simulink model "doublePendulum"  (R2022a)
settings: Solver=ode45  StartTime=0.0  StopTime=50  MaxStep=0.001  RelTol=1e-4
undefined symbols (not defined in the file): a_x, a_y, omega_x, omega_y
settings Model: Creator=semen  LastModifiedBy=semen

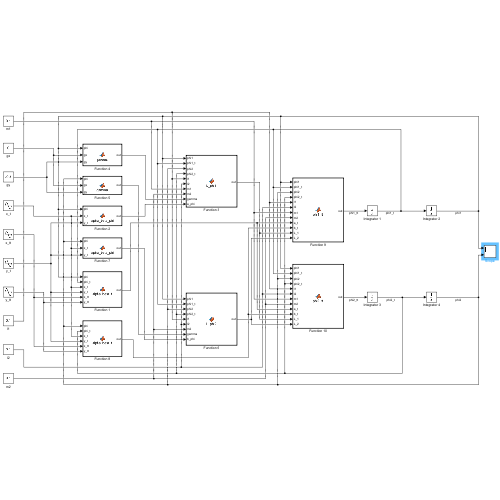
[thumbnail: Simulink's stored preview of the top-level diagram]
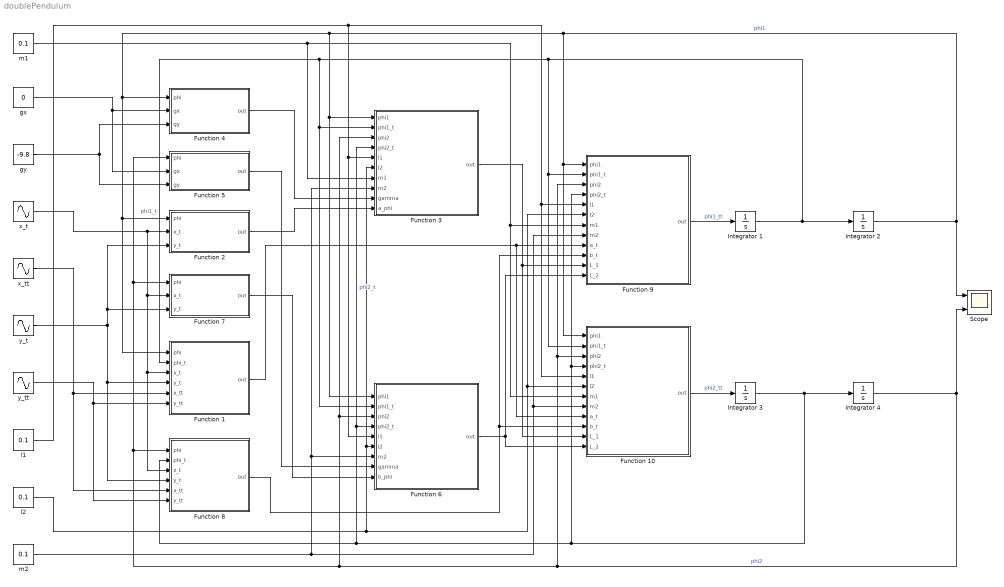
== system doublePendulum ==
  Function 1 : MATLAB Function  TreatAsAtomicUnit=on
  Function 10 : MATLAB Function  TreatAsAtomicUnit=on
  Function 2 : MATLAB Function  TreatAsAtomicUnit=on
  Function 3 : MATLAB Function  TreatAsAtomicUnit=on
  Function 4 : MATLAB Function  TreatAsAtomicUnit=on
  Function 5 : MATLAB Function  TreatAsAtomicUnit=on
  Function 6 : MATLAB Function  TreatAsAtomicUnit=on
  Function 7 : MATLAB Function  TreatAsAtomicUnit=on
  Function 8 : MATLAB Function  TreatAsAtomicUnit=on
  Function 9 : MATLAB Function  TreatAsAtomicUnit=on
  Integrator 1 : Integrator
  Integrator 2 : Integrator  InitialCondition=pi / 2
  Integrator 3 : Integrator
  Integrator 4 : Integrator  InitialCondition=pi / 2
  Scope : Scope  NumInputPorts=2
  gx : Constant  Value=0
  gy : Constant  Value=-9.8
  l1 : Constant  Value=0.1
  l2 : Constant  Value=0.1
  m1 : Constant  Value=0.1
  m2 : Constant  Value=0.1
  x_t : Sin  Amplitude=a_x * omega_x  Frequency=omega_x  Phase=pi / 2  SampleTime=0
  x_tt : Sin  Amplitude=-a_x * omega_x ^ 2  Frequency=omega_x  SampleTime=0
  y_t : Sin  Amplitude=a_y * omega_y  Frequency=omega_y  Phase=pi / 2  SampleTime=0
  y_tt : Sin  Amplitude=-a_y * omega_y ^ 2  Frequency=omega_y  SampleTime=0
  wires:
  Integrator 1/1 -> Function 10/2(phi1_t), Function 9/2(phi1_t), Function 1/2(phi_t), Function 6/2(phi1_t), Function 3/2(phi1_t), Integrator 2/1  "phi1_t"
  Integrator 2/1 -> Function 10/1(phi1), Function 9/1(phi1), Function 6/1(phi1), Function 3/1(phi1), Function 1/1(phi), Function 2/1(phi), Function 4/1(phi), Scope/1  "phi1"
  Function 9/1(out) -> Integrator 1/1  "phi1_tt"
  Function 10/1(out) -> Integrator 3/1  "phi2_tt"
  Integrator 3/1 -> Integrator 4/1, Function 8/2(phi_t), Function 3/4(phi2_t), Function 6/4(phi2_t), Function 9/4(phi2_t), Function 10/4(phi2_t)  "phi2_t"
  Integrator 4/1 -> Scope/2, Function 9/3(phi2), Function 10/3(phi2), Function 8/1(phi), Function 7/1(phi), Function 5/1(phi), Function 3/3(phi2), Function 6/3(phi2)  "phi2"
  gx/1 -> Function 5/2(gx), Function 4/2(gx)
  gy/1 -> Function 4/3(gy), Function 5/3(gy)
  x_t/1 -> Function 7/2(x_t), Function 1/3(x_t), Function 8/3(x_t), Function 2/2(x_t)
  y_t/1 -> Function 2/3(y_t), Function 7/3(y_t), Function 8/4(y_t), Function 1/4(y_t)
  x_tt/1 -> Function 8/5(x_tt), Function 1/5(x_tt)
  y_tt/1 -> Function 1/6(y_tt), Function 8/6(y_tt)
  l1/1 -> Function 6/5(l1), Function 3/5(l1), Function 10/5(l1), Function 9/5(l1)
  l2/1 -> Function 3/6(l2), Function 6/6(l2), Function 9/6(l2), Function 10/6(l2)
  m1/1 -> Function 3/7(m1), Function 10/7(m1), Function 9/7(m1)
  m2/1 -> Function 9/8(m2), Function 10/8(m2), Function 3/8(m2), Function 6/7(m2)
  Function 4/1(out) -> Function 3/9(gamma)
  Function 5/1(out) -> Function 6/8(gamma)
  Function 2/1(out) -> Function 3/10(a_phi)
  Function 7/1(out) -> Function 6/9(b_phi)
  Function 1/1(out) -> Function 10/9(a_t), Function 9/9(a_t)
  Function 8/1(out) -> Function 9/10(b_t), Function 10/10(b_t)
  Function 3/1(out) -> Function 10/11(L_1), Function 9/11(L_1)
  Function 6/1(out) -> Function 10/12(L_2), Function 9/12(L_2)

== matlab function doublePendulum/Function 8 ==
  data: phi input; out output; phi_t input; x_t input; y_t input; x_tt input; y_tt input
function out = alpha_beta_t(phi, phi_t, x_t, y_t, x_tt, y_tt)
    out = cos(phi) * (x_tt + y_t * phi_t) + ...
        sin(phi) * (y_tt - x_t * phi_t);
end

== matlab function doublePendulum/Function 9 ==
  data: phi1 input; out output; phi1_t input; phi2 input; phi2_t input; l1 input; l2 input; m1 input; m2 input; a_t input; b_t input; L_1 input; L_2 input
function out = phi1_tt(phi1, phi1_t, phi2, phi2_t, l1, l2, m1, m2, a_t, ...
    b_t, L_1, L_2)
    delta = phi2 - phi1;
    out = (L_1 / l1 ^ 2 - L_2 * cos(delta) / l1 / l2 - ...
        m2 / l1 * sin(delta) * (phi2_t - phi1_t) * ...
        (l1 * cos(delta) * phi1_t - l2 * phi2_t) - ...
        ((m1 + m2) * a_t - m2 * cos(delta) * b_t) / l1) / ...
        (m1 + m2 * sin(delta) ^ 2);
end

== matlab function doublePendulum/Function 10 ==
  data: phi1 input; out output; phi1_t input; phi2 input; phi2_t input; l1 input; l2 input; m1 input; m2 input; a_t input; b_t input; L_1 input; L_2 input
function out = phi2_tt(phi1, phi1_t, phi2, phi2_t, l1, l2, m1, m2, ...
    a_t, b_t, L_1, L_2)
    delta = phi2 - phi1;
    out = (L_2 * (m1 + m2) / m2 / l2 ^ 2 - L_1 * cos(delta) / l1 / l2 - ...
        sin(delta) * (phi2_t - phi1_t) / l2 * ...
        (m2 * l2 * cos(delta) * phi2_t - (m1 + m2) * l1 * phi1_t) - ...
        (b_t - cos(delta) * a_t) * (m1 + m2) / l2) / ...
        (m1 + m2 * sin(delta) ^ 2);
end

== matlab function doublePendulum/Function 1 ==
  data: phi input; out output; phi_t input; x_t input; y_t input; x_tt input; y_tt input
function out = alpha_beta_t(phi, phi_t, x_t, y_t, x_tt, y_tt)
    out = cos(phi) * (x_tt + y_t * phi_t) + ...
        sin(phi) * (y_tt - x_t * phi_t);
end

== matlab function doublePendulum/Function 2 ==
  data: phi input; out output; x_t input; y_t input
function out = alpha_beta_phi(phi, x_t, y_t)
    out = cos(phi) * y_t - sin(phi) * x_t;
end

== matlab function doublePendulum/Function 3 ==
  data: phi1 input; out output; phi1_t input; phi2 input; phi2_t input; l1 input; l2 input; m1 input; m2 input; gamma input; a_phi input
function out = L_phi1(phi1, phi1_t, phi2, phi2_t, l1, l2, ...
    m1, m2, gamma, a_phi)
    out = phi1_t * l1 * (m1 + m2) * a_phi + m2 * l1 * l2 * phi1_t * ...
        phi2_t * sin(phi2 - phi1) + (m1 + m2) * l1 * gamma;
end

== matlab function doublePendulum/Function 4 ==
  data: phi input; out output; gx input; gy input
function out = gamma(phi, gx, gy)
    out = cos(phi) * gx + sin(phi) * gy;
end

== matlab function doublePendulum/Function 5 ==
  data: phi input; out output; gx input; gy input
function out = gamma(phi, gx, gy)
    out = cos(phi) * gx + sin(phi) * gy;
end

== matlab function doublePendulum/Function 6 ==
  data: phi1 input; out output; phi1_t input; phi2 input; phi2_t input; l1 input; l2 input; m2 input; gamma input; b_phi input
function out = L_phi2(phi1, phi1_t, phi2, phi2_t, l1, l2, m2, gamma, b_phi)
    out = phi2_t * l2 * m2 * b_phi - m2 * l1 * l2 * phi1_t * ...
        phi2_t * sin(phi2 - phi1) + m2 * l2 * gamma;
end

== matlab function doublePendulum/Function 7 ==
  data: phi input; out output; x_t input; y_t input
function out = alpha_beta_phi(phi, x_t, y_t)
    out = cos(phi) * y_t - sin(phi) * x_t;
end
